simulink model "TV_2018_HIL"  (R2016a)
settings: Solver=FixedStepAuto  StartTime=0.0  StopTime=inf  FixedStep=0.001  RelTol=1e-3
PreLoadFcn:
  | TV_2017_parameters
values from neighbouring files (symbols this model uses):
  battery_voltage = single(530)    [HIL_parameters.m]    (also in HIL_parameters_2018.m; TV_2017_parameters.m; TV_2017_parameters_VD.m)
  car_params = Simulink_Car_params    [HIL_parameters.m]    (also in HIL_parameters_2018.m; TV_2017_parameters.m; TV_2017_parameters_VD.m)
  i_Diff = 16    [HIL_parameters.m]    (also in HIL_parameters_2018.m; TV_2017_parameters.m)
  Kp = 1    [HIL_parameters.m]    (also in HIL_parameters_2018.m; TV_2017_parameters.m; TV_2017_parameters_VD.m)
  motor_data = struct    [HIL_parameters.m]    (also in HIL_parameters_2018.m; TV_2017_parameters.m)
  powerLimitControl = Simulink_el    [HIL_parameters.m]    (also in HIL_parameters_2018.m; TV_2017_parameters.m; TV_2017_parameters_VD.m)
  settings = Simulink_Settings    [HIL_parameters.m]    (also in HIL_parameters_2018.m; TV_2017_parameters.m; TV_2017_parameters_VD.m)
  SpdC_BCC = 0    [HIL_parameters.m]    (also in HIL_parameters_2018.m; TV_2017_parameters.m; TV_2017_parameters_VD.m)
  Speed_Neg_sat = -21    [HIL_parameters.m]    (also in HIL_parameters_2018.m; TV_2017_parameters.m; TV_2017_parameters_VD.m)
  Speed_Pos_sat = 21    [HIL_parameters.m]    (also in HIL_parameters_2018.m; TV_2017_parameters.m; TV_2017_parameters_VD.m)
  SteeringAngleFL = [-23.80 -22.65 -21.50 -20.34 -19.18 -18.03 -16.86 -15.70 -14.53 -13.35 -12.18 -10.99 -9.80 -8.61 -7.40 -6.19 -4.97 -3.75 -2.51 -1.26 0 1.27 2.56 3.85 5.17 6.50 7.84 9.21 10.59 12.00 13.42 14.88 16.36 17.87 19.41 20.99 22.61 24.26 25.97 27.73 29.54]    [CarSetupAnalysis2018.m]    (also in HIL_parameters_2018.m; TV_2017_parameters.m; TV_2017_parameters_VD.m = [-24.129 -22.950 -21.772 -20.593 -19.413 -18.232 -17.050 -15)
  SteeringAngleFR = [-29.54 -27.73 -25.97 -24.26 -22.61 -20.99 -19.41 -17.87 -16.36 -14.88 -13.42 -12.00 -10.59 -9.21 -7.84 -6.50 -5.17 -3.85 -2.56 -1.27 0 1.26 2.51 3.75 4.97 6.19 7.40 8.61 9.80 10.99 12.18 13.35 14.53 15.70 16.86 18.03 19.18 20.34 21.50 22.65 23.80]    [CarSetupAnalysis2018.m]    (also in HIL_parameters_2018.m; TV_2017_parameters.m; TV_2017_parameters_VD.m = [-29.3050 -27.5340 -25.8140 -24.1410 -22.5110 -20.9180 -19.3)
  SteeringWhAngle = [-105 -99.75 -94.5 -89.25 -84 -78.75 -73.5 -68.25 -63 -57.75 -52.5 -47.25 -42 -36.75 -31.5 -26.25 -21.0 -15.75 -10.5 -5.25 0.0 5.25 10.50 15.75 21.00 26.25 31.50 36.75 42.00 47.25 52.50 57.75  63.00 68.25 73.50 78.75 84.00 89.25 94.50 99.75 105.00]    [TV_2017_parameters_VD.m]
  Tn_n = 0    [HIL_parameters.m]    (also in HIL_parameters_2018.m; TV_2017_parameters.m; TV_2017_parameters_VD.m)
  tractionControl = Simulink_tc    [HIL_parameters.m]    (also in HIL_parameters_2018.m; IterativeTractionControlTuning.m; TV_2017_parameters.m; TV_2017_parameters_VD.m)
  yawMomentGenerator = struct    [HIL_parameters.m]    (also in HIL_parameters_2018.m = Simulink_yawRate2; TV_2017_parameters.m = Simulink_yawRate2)
  yawRateControl = Simulink_yawRate    [HIL_parameters.m]    (also in HIL_parameters_2018.m; TV_2017_parameters.m; TV_2017_parameters_VD.m)
undefined symbols (not defined in the file or in its folder): canChannel, DiscIntNeverNeededParam, magnitude, speedEstimation, TC_Decr_Gas, TC_Derivative, TC_Incr_Gas, TC_On, TC_Relay_Off, TC_Relay_On
libraries: CarMaker4SL x366, simulink_extras x63, canmsglib x55, canlib x41, simulink x37, dspfdesign x2, sldrtlib x1
(part 1 of 15)
settings Model: Creator=fh  LastModifiedBy=95fre
settings DataIOCC: LimitDataPoints=on  SaveFormat=Array  SignalLoggingSaveFormat=ModelDataLogs  SignalLoggingName=sigsOut
settings OptimizationCC: DefaultUnderspecifiedDataType=single  OptimizeBlockIOStorage=off  BufferReuse=off  GlobalBufferReuse=off  ExpressionFolding=off  ExpressionDepthLimit=2147483647  LocalBlockOutputs=off  OptimizeModelRefInitCode=on  LifeSpan=Inf  MaxStackSize=64
settings DebuggingCC: SaveWithParameterizedLinksMsg=none  UnderspecifiedInitializationDetection=Classic  SignalResolutionControl=TryResolveAllWithWarning  MultiTaskDSMMsg=warning  MultiTaskCondExecSysMsg=none  BusObjectLabelMismatch=error  ModelReferenceVersionMismatchMessage=warning  StateNameClashWarn=warning
settings HardwareCC: ProdBitPerPointer=32  ProdLargestAtomicInteger=Long  ProdLargestAtomicFloat=Double  ProdWordSize=32  ProdHWDeviceType=ARM Compatible->ARM Cortex  TargetLargestAtomicInteger=Long  TargetLargestAtomicFloat=Double  TargetEndianess=LittleEndian  TargetHWDeviceType=ARM Compatible->ARM Cortex
settings ModelReferenceCC: PropagateSignalLabelsOutOfModel=off
settings RTWCC: SystemTargetFile=ert.tlc  GenCodeOnly=on  TemplateMakefile=ert_default_tmf  GenerateReport=on  Toolchain=GNU Tools for ARM Embedded Processors  BuildConfiguration=Debug  IncludeHyperlinkInReport=on  LaunchReport=on
settings CodeAppCC: ForceParamTrailComments=on  IgnoreCustomStorageClasses=off  SimulinkDataObjDesc=on  SFDataObjDesc=on  MATLABFcnDesc=on  InsertBlockDesc=on  MATLABSourceComments=on  EnableCustomComments=on  ReqsInCode=on
settings ERTTargetCC: GenerateSampleERTMain=on  IncludeMdlTerminateFcn=off  MatFileLogging=on  SupportNonFinite=off  SupportComplex=off  SupportVariableSizeSignals=on  ERTCustomFileTemplate=example_file_process.tlc  SuppressUnreachableDefaultCases=off
settings ConfigComp: CovHTMLOptions=-sRT=1 -sVT=0 -aTS=1 -bRG=1 -bTC=1 -hTR=0 -nFC=0 -nFD=1 -scm=1 -bcm=1 -xEv=0 -xEM=0  CovModelRefEnable=Off  PSAutoStubLUT=off

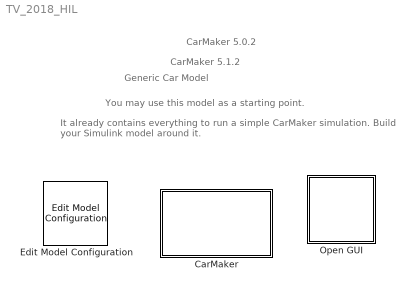
== system TV_2018_HIL ==
  note: Generic Car Model
  note: You may use this model as a starting point.
  note: It already contains everything to run a simple CarMaker simulation.
      | Build your Simulink model around it.
  note: CarMaker 5.0.2
  note: CarMaker 5.1.2
  CarMaker : Subsystem  TreatAsAtomicUnit=on
      mask Display: image(imread('CarMakerSys.png'));
  Edit Model Configuration : CarMaker4SL/Edit Model Configuration
  Open GUI : Subsystem  LoadFcn=if ~length(which('cmcmd')), cmenv; end
      settings: OpenFcn=cmblockmagic('gui_fix_display'); CM_Simulink
      mask Display: image('CarMakerGUI.png');

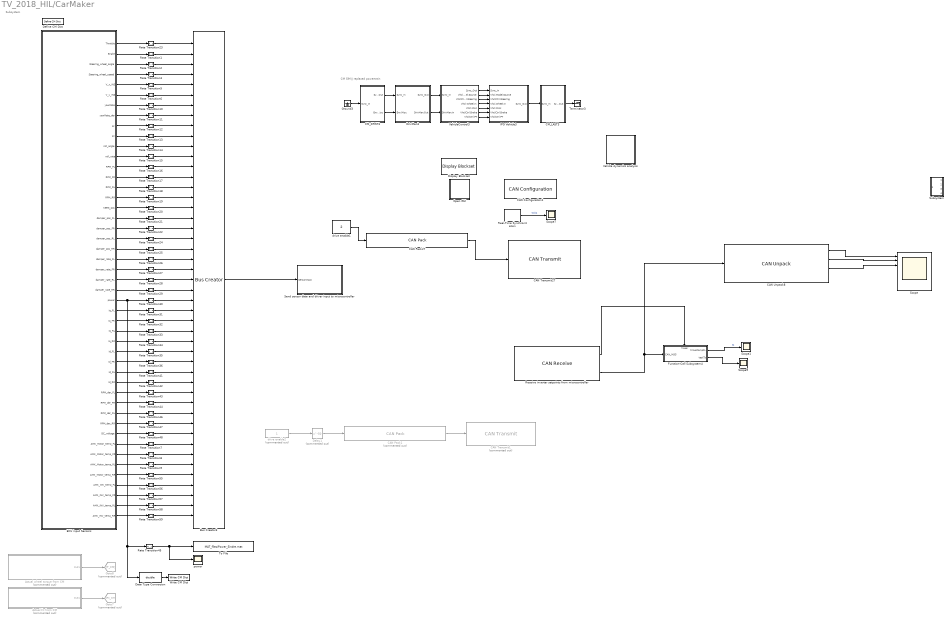
== system TV_2018_HIL/CarMaker ==
  note: Subsystem
  note: CM SIM|| replaced powertrain
  Actual Fz from CM : Subsystem  Commented=on
  Actual wheel torque from CM : Subsystem  Commented=on
  Bus Creator3 : BusCreator  Inputs=47  OutDataTypeStr=Bus: SensorInputs  NonVirtualBus=on
      settings: InheritFromInputs=off
  CAN Configuration1 : canlib/CAN Configuration  BlockHandle=108.0002  DeviceMenu=Kvaser Virtual 1 (Channel 1)  Device=PEAK-System PCAN-USB (PCAN_USBBUS1)  ObjConstructor=canChannel('PEAK-System', 'PCAN_PCIBUS1')  BusSpeed=1000000  EnableBitParameters=off  SJW=NaN  TSEG1=NaN  TSEG2=NaN  NSamples=NaN  AckMode=Normal
  CAN Pack1 : canmsglib/CAN Pack  Commented=on  MsgList=(none)  MsgName=CAN Msg  MsgIDType=Standard (11-bit identifier)  MsgIdentifier=DRIVE_ENABLE  MsgLength=0  NSignals=0  StartBits=0  SignalSizes=0  ByteOrders=0  DataTypes=0  MultiplexTypes=0  MultiplexValues=0  Factors=0  Offsets=0  Minimums=0  Maximums=0  Remote=off
      settings: DataFormat=manually specified signals
  CAN Pack27 : canmsglib/CAN Pack  MsgList=(none)  MsgName=CAN Msg  MsgIDType=Standard (11-bit identifier)  MsgIdentifier=BMS_STATE  MsgLength=4  NSignals=0  StartBits=0  SignalSizes=0  ByteOrders=0  DataTypes=0  MultiplexTypes=0  MultiplexValues=0  Factors=0  Offsets=0  Minimums=0  Maximums=0  Remote=off
      settings: DataFormat=raw data
  CAN Transmit1 : canlib/CAN Transmit  Commented=on  BlockHandle=111.0002  DeviceMenu=Kvaser Virtual 1 (Channel 1)  Device=PEAK-System PCAN-USB (PCAN_USBBUS1)  ObjConstructor=canChannel('PEAK-System', 'PCAN_PCIBUS1')  EnablePeriodicTransmit=off  MessagePeriod=1.000
  CAN Transmit27 : canlib/CAN Transmit  BlockHandle=112.0002  DeviceMenu=Kvaser Virtual 1 (Channel 1)  Device=PEAK-System PCAN-USB (PCAN_USBBUS1)  ObjConstructor=canChannel('PEAK-System', 'PCAN_PCIBUS1')  EnablePeriodicTransmit=off  MessagePeriod=1.000
  CAN Unpack8 : canmsglib/CAN Unpack  MsgList=(none)  MsgName=TestTimestamp  MsgIDType=Standard (11-bit identifier)  MsgIdentifier=ECU_STATE  MsgLength=4  SignalInfo=sys_state$0$16$1$2$1$0$1$0$-Inf$Inf$#Torque_Alloc$16$8$1$2$1$0$1$0$-Inf$Inf$#Vehicle_state$24$8$1$2$1$0$1$0$-Inf$Inf$#  NSignals=3  IDPort=off  TimestampPort=on  ErrorPort=off  RemotePort=off  LengthPort=off  StatusPort=off  StartBits=str2num('[int32(0);int32(16);int32(24)]')  SignalSizes=str2num('[int32(16);int32(8);int32(8)]')  ByteOrders=str2num('[int32(1);int32(1);int32(1)]')  DataTypes=str2num('[int32(2);int32(2);int32(2)]')  MultiplexTypes=str2num('[int32(1);int32(1);int32(1)]')  MultiplexValues=str2num('[double(0);double(0);double(0)]')  Factors=str2num('[double(1);double(1);double(1)]')  Offsets=str2num('[double(0);double(0);double(0)]')  Minimums=str2num('[double(-Inf);double(-Inf);double(-Inf)]')  Maximums=str2num('[double(Inf);double(Inf);double(Inf)]')
  CM_FIRST3 : Subsystem
  CM_LAST3 : Subsystem
  Data Type Conversion : DataTypeConversion  OutDataTypeStr=double
  Define CM Dict : CarMaker4SL/Define CM Dict  xname=Power  xmono=off  xtype=Double  xdvaplace=None  xnstates=0  xfirststate=0  xinitial=0
  Delay1 : Delay  Commented=on  DelayLength=50
  Display Blockset : CarMaker4SL/Display Blockset
  DrivMan3 : Subsystem
  "ECU input Sensors " : Subsystem  SystemSampleTime=settings.control_system_sample_time
  Function-Call Subsystem4 : Subsystem  TreatAsAtomicUnit=on
  Goto7 : Goto  Commented=on  GotoTag=Fz_CM
  Goto8 : Goto  Commented=on  GotoTag=T_CM
  Ground3 : Ground
  IPG Vehicle3 : Subsystem  TreatAsAtomicUnit=on
  Open GUI : Subsystem  LoadFcn=if ~length(which('cmcmd')), cmenv; end
      settings: OpenFcn=cmblockmagic('gui_fix_display'); CM_Simulink
      mask Display: image('CarMakerGUI.png');
  Rate Transition{1..3,5..36,41..48,55..59} (48 alike) : RateTransition  OutPortSampleTime=matlab_params.sensor_sampling_time
  Real-Time Synchronization : sldrtlib/Real-Time Synchronization  SampleTime=0.01  MaxMissedTicks=100000  ShowMissedTicks=on  YieldWhenWaiting=on
  Receive inverter setpoints from microcontroller : canlib/CAN Receive  BlockHandle=19018.001  DeviceMenu=Kvaser Virtual 1 (Channel 1)  Device=PEAK-System PCAN-USB (PCAN_USBBUS1)  ObjConstructor=canChannel('PEAK-System', 'PCAN_PCIBUS1')  EnableStandardIDsFilter=off  StandardIDs=listen_ID  EnableExtendedIDsFilter=off  ExtendedIDs=0  SampleTime=0.001  MsgsPerTimestep=all  StdIDsCombo=Allow all  ExtIDsCombo=Allow all  InternalFilterUpdateStatus=on
  Scope : Scope  NumInputPorts=8
  Scope1 : Scope
  Scope7 : Scope
  Scope9 : Scope
  "Send sensor data and driver input to microcontroller " : Subsystem
  Subsystem : Subsystem
  Terminator3 : Terminator
  To File : ToFile  Filename=MAT_files\Power_Sindre.mat  MatrixName=Power  SaveFormat=Timeseries
  Vehicle dynamics analysis : Subsystem
  VehicleControl3 : Subsystem
  Write CM Dict : CarMaker4SL/Write CM Dict  xname=Power  xsync=off
  drive enable1 : Constant  Value=2  OutDataTypeStr=uint8
  drive enable2 : Constant  Commented=on
  power : Scope
  wires:
  VehicleControl3/7(VhclCtrl.PT) -> IPG Vehicle3/7(VhclCtrl.PT)
  VehicleControl3/6(VhclCtrl.Brake) -> IPG Vehicle3/6(VhclCtrl.Brake)
  CM_FIRST3/1(Sync_Out) -> DrivMan3/1(Sync_In)
  CM_FIRST3/2(Env.Misc) -> DrivMan3/2(Env.Misc)
  VehicleControl3/3(VhclCtrl.Steering) -> IPG Vehicle3/3(VhclCtrl.Steering)
  DrivMan3/2(DrivMan.Out) -> VehicleControl3/2(DrivMan.In)
  VehicleControl3/2(Vhcl.Model.Source) -> IPG Vehicle3/2(Vhcl.Model.Source)
  VehicleControl3/5(Vhcl.Misc) -> IPG Vehicle3/5(Vhcl.Misc)
  VehicleControl3/1(Sync_Out) -> IPG Vehicle3/1(Sync_In)
  VehicleControl3/4(Vhcl.Wheel.In) -> IPG Vehicle3/4(Vhcl.Wheel.In)
  DrivMan3/1(Sync_Out) -> VehicleControl3/1(Sync_In)
  Ground3/1 -> CM_FIRST3/1(Sync_In)
  IPG Vehicle3/1(Sync_Out) -> CM_LAST3/1(Sync_In)
  CM_LAST3/1(Sync_Out) -> Terminator3/1
  Receive inverter setpoints from microcontroller/1 -> Function-Call Subsystem4/Trigger
  Function-Call Subsystem4/1(timestampFL) -> Scope1/1  "ts"
  Function-Call Subsystem4/2(testTs) -> Scope9/1
  Real-Time Synchronization/1 -> Scope7/1  "ticks"
  Rate Transition9/1 -> Bus Creator3/42
  Rate Transition7/1 -> Bus Creator3/40
  Rate Transition27/1 -> Bus Creator3/23
  "ECU input Sensors "/40(AMK_Motor_temp_FL) -> Rate Transition7/1
  "ECU input Sensors "/46(AMK_INV_temp_RL) -> Rate Transition58/1
  "ECU input Sensors "/41(AMK_Motor_temp_FR) -> Rate Transition8/1
  Rate Transition10/1 -> Bus Creator3/7
  Rate Transition46/1 -> Bus Creator3/37
  "ECU input Sensors "/44(AMK_INV_temp_FL) -> Rate Transition56/1
  Rate Transition5/1 -> Bus Creator3/5
  Actual Fz from CM/1(Out1) -> Goto7/1
  "ECU input Sensors "/42(AMK_Motor_temp_RL) -> Rate Transition9/1
  "ECU input Sensors "/26(power) -> Data Type Conversion/1, Rate Transition45/1, Rate Transition30/1
  Rate Transition58/1 -> Bus Creator3/46
  Rate Transition32/1 -> Bus Creator3/28
  Rate Transition57/1 -> Bus Creator3/45
  Rate Transition47/1 -> Bus Creator3/38
  "ECU input Sensors "/43(AMK_Motor_temp_RR) -> Rate Transition55/1
  Rate Transition48/1 -> Bus Creator3/39
  Rate Transition19/1 -> Bus Creator3/16
  Actual wheel torque from CM/1(Out1) -> Goto8/1
  Rate Transition13/1 -> Bus Creator3/10
  Rate Transition59/1 -> Bus Creator3/47
  Rate Transition56/1 -> Bus Creator3/44
  "ECU input Sensors "/47(AMK_INV_temp_RR) -> Rate Transition59/1
  Rate Transition55/1 -> Bus Creator3/43
  Rate Transition33/1 -> Bus Creator3/29
  "ECU input Sensors "/45(AMK_INV_temp_FR) -> Rate Transition57/1
  Data Type Conversion/1 -> Write CM Dict/1
  Rate Transition41/1 -> Bus Creator3/33
  Rate Transition34/1 -> Bus Creator3/30
  Rate Transition43/1 -> Bus Creator3/35
  Rate Transition42/1 -> Bus Creator3/34
  Rate Transition44/1 -> Bus Creator3/36
  Rate Transition8/1 -> Bus Creator3/41
  Rate Transition36/1 -> Bus Creator3/32
  Rate Transition35/1 -> Bus Creator3/31
  Rate Transition6/1 -> Bus Creator3/6
  Rate Transition28/1 -> Bus Creator3/24
  Rate Transition21/1 -> Bus Creator3/18
  "ECU input Sensors "/32(Id_FR) -> Rate Transition36/1
  "ECU input Sensors "/3("Steering_wheel_angle ") -> Rate Transition2/1
  "ECU input Sensors "/34(Id_RR) -> Rate Transition42/1
  "ECU input Sensors "/7(yawRate) -> Rate Transition10/1
  "ECU input Sensors "/31(Id_FL) -> Rate Transition35/1
  "ECU input Sensors "/1("Throttle ") -> Rate Transition23/1
  Rate Transition26/1 -> Bus Creator3/22
  Rate Transition31/1 -> Bus Creator3/27
  "ECU input Sensors "/13(RPM_FL) -> Rate Transition16/1
  Rate Transition18/1 -> Bus Creator3/15
  Rate Transition11/1 -> Bus Creator3/8
  Rate Transition14/1 -> Bus Creator3/11
  Rate Transition30/1 -> Bus Creator3/26
  "ECU input Sensors "/16(RPM_RR) -> Rate Transition19/1
  Rate Transition23/1 -> Bus Creator3/1
  "ECU input Sensors "/6(V_y_INS) -> Rate Transition6/1
  "ECU input Sensors "/24(damper_rate_RL) -> Rate Transition28/1
  "ECU input Sensors "/19(damper_pos_FR) -> Rate Transition22/1
  "ECU input Sensors "/29(Iq_RL) -> Rate Transition33/1
  "ECU input Sensors "/25(damper_rate_RR) -> Rate Transition29/1
  "ECU input Sensors "/5(V_x_INS) -> Rate Transition5/1
  Rate Transition2/1 -> Bus Creator3/3
  Rate Transition17/1 -> Bus Creator3/14
  "ECU input Sensors "/30(Iq_RR) -> Rate Transition34/1
  "ECU input Sensors "/12(roll_rate) -> Rate Transition15/1
  "ECU input Sensors "/22(damper_rate_FL) -> Rate Transition26/1
  "ECU input Sensors "/28(Iq_FR) -> Rate Transition32/1
  "ECU input Sensors "/11(roll_angle) -> Rate Transition14/1
  "ECU input Sensors "/2("Brake ") -> Rate Transition1/1
  "ECU input Sensors "/17(KERS_pos) -> Rate Transition20/1
  Rate Transition15/1 -> Bus Creator3/12
  Rate Transition29/1 -> Bus Creator3/25
  Rate Transition24/1 -> Bus Creator3/20
  Rate Transition1/1 -> Bus Creator3/2
  Rate Transition20/1 -> Bus Creator3/17
  Rate Transition12/1 -> Bus Creator3/9
  "ECU input Sensors "/20(damper_pos_RL) -> Rate Transition24/1
  "ECU input Sensors "/15(RPM_RL) -> Rate Transition18/1
  Rate Transition22/1 -> Bus Creator3/19
  Rate Transition3/1 -> Bus Creator3/4
  Rate Transition25/1 -> Bus Creator3/21
  "ECU input Sensors "/10("ax ") -> Rate Transition13/1
  Rate Transition16/1 -> Bus Creator3/13
  "ECU input Sensors "/39(DC_voltage) -> Rate Transition48/1
  "ECU input Sensors "/18(damper_pos_FL) -> Rate Transition21/1
  "ECU input Sensors "/8(yawRate_der) -> Rate Transition11/1
  "ECU input Sensors "/4(Steering_wheel_speed) -> Rate Transition3/1
  "ECU input Sensors "/27(Iq_FL) -> Rate Transition31/1
  "ECU input Sensors "/14(RPM_FR) -> Rate Transition17/1
  "ECU input Sensors "/21(damper_pos_RR) -> Rate Transition25/1
  "ECU input Sensors "/9(ay) -> Rate Transition12/1
  "ECU input Sensors "/33(Id_RL) -> Rate Transition41/1
  "ECU input Sensors "/23(damper_rate_FR) -> Rate Transition27/1
  Rate Transition45/1 -> power/1, To File/1
  "ECU input Sensors "/35(RPM_der_FL) -> Rate Transition43/1
  "ECU input Sensors "/36(RPM_der_FR) -> Rate Transition44/1
  "ECU input Sensors "/38(RPM_der_RR) -> Rate Transition47/1
  "ECU input Sensors "/37(RPM_der_RL) -> Rate Transition46/1
  CAN Pack27/1 -> CAN Transmit27/1
  Receive inverter setpoints from microcontroller/2 -> CAN Unpack8/1, Function-Call Subsystem4/1(CAN_MSG)
  CAN Unpack8/1 -> Scope/1
  CAN Unpack8/2 -> Scope/2
  CAN Unpack8/3 -> Scope/3
  drive enable1/1 -> CAN Pack27/1
  CAN Pack1/1 -> CAN Transmit1/1
  drive enable2/1 -> Delay1/1
  Delay1/1 -> CAN Pack1/1
  Bus Creator3/1 -> "Send sensor data and driver input to microcontroller "/1(SensorInput)

== system TV_2018_HIL/Open GUI ==
  S-Function : S-Function  FunctionName=cm_gui  SFunctionDeploymentMode=off  EnableBusSupport=off

== system TV_2018_HIL/CarMaker/Actual Fz from CM ==
  Bus Creator1 : BusCreator  Inputs=4
  Bus Creator4 : BusCreator  Inputs=4  OutDataTypeStr=Bus: normalForces  NonVirtualBus=on
      settings: InheritFromInputs=off
  Data Type Conversion{4..11} (8 alike) : DataTypeConversion  OutDataTypeStr=single
  Divide{,1..3} (4 alike) : Product  Inputs=*/
  Friction : Scope
  Rate Transition4 : RateTransition  OutPortSampleTime=matlab_params.sensor_sampling_time
  Read CM Dict10 : CarMaker4SL/Read CM Dict  xname=Vhcl.RL.Fx  xsync=off
  Read CM Dict11 : CarMaker4SL/Read CM Dict  xname=Vhcl.RR.Fx  xsync=off
  Read CM Dict3 : CarMaker4SL/Read CM Dict  xname=Vhcl.FR.Fz  xsync=off
  Read CM Dict4 : CarMaker4SL/Read CM Dict  xname=Vhcl.FL.Fz  xsync=off
  Read CM Dict5 : CarMaker4SL/Read CM Dict  xname=Vhcl.RR.Fz  xsync=off
  Read CM Dict6 : CarMaker4SL/Read CM Dict  xname=Vhcl.RL.Fz  xsync=off
  Read CM Dict8 : CarMaker4SL/Read CM Dict  xname=Vhcl.FL.Fx  xsync=off
  Read CM Dict9 : CarMaker4SL/Read CM Dict  xname=Vhcl.FR.Fx  xsync=off
  Out1 : Outport
  wires:
  Rate Transition4/1 -> Out1/1
  Read CM Dict4/1 -> Data Type Conversion4/1
  Read CM Dict5/1 -> Data Type Conversion7/1
  Read CM Dict3/1 -> Data Type Conversion5/1
  Read CM Dict6/1 -> Data Type Conversion6/1
  Data Type Conversion7/1 -> Bus Creator4/4, Divide3/2
  Data Type Conversion5/1 -> Bus Creator4/2, Divide1/2
  Data Type Conversion6/1 -> Bus Creator4/3, Divide2/2
  Divide/1 -> Bus Creator1/1  "FL"
  Read CM Dict10/1 -> Data Type Conversion10/1
  Data Type Conversion11/1 -> Divide3/1
  Data Type Conversion9/1 -> Divide1/1
  Data Type Conversion8/1 -> Divide/1
  Read CM Dict9/1 -> Data Type Conversion9/1
  Read CM Dict11/1 -> Data Type Conversion11/1
  Divide3/1 -> Bus Creator1/4  "RR"
  Bus Creator1/1 -> Friction/1
  Data Type Conversion4/1 -> Bus Creator4/1, Divide/2
  Read CM Dict8/1 -> Data Type Conversion8/1
  Divide2/1 -> Bus Creator1/3  "RL"
  Bus Creator4/1 -> Rate Transition4/1
  Data Type Conversion10/1 -> Divide2/1
  Divide1/1 -> Bus Creator1/2  "FR"

== system TV_2018_HIL/CarMaker/Actual wheel torque from CM ==
  Bus Creator2 : BusCreator  Inputs=4  OutDataTypeStr=Bus: T_meas
      settings: InheritFromInputs=off
  Data Type Conversion{1..3,12..15} (7 alike) : DataTypeConversion  OutDataTypeStr=single
  Rate Transition{37..40} (4 alike) : RateTransition  OutPortSampleTime=matlab_params.sensor_sampling_time
  Read CM Dict1 : CarMaker4SL/Read CM Dict  xname=Car.DampFL.Frc_tot  xsync=off
  Read CM Dict12 : CarMaker4SL/Read CM Dict  xname=PT.WFL.Trq_Drive  xsync=off
  Read CM Dict2 : CarMaker4SL/Read CM Dict  xname=Car.SpringFL.Frc_tot  xsync=off
  Read CM Dict45 : CarMaker4SL/Read CM Dict  xname=PT.WFR.Trq_Drive  xsync=off
  Read CM Dict46 : CarMaker4SL/Read CM Dict  xname=PT.WRL.Trq_Drive  xsync=off
  Read CM Dict47 : CarMaker4SL/Read CM Dict  xname=PT.WRR.Trq_Drive  xsync=off
  Read CM Dict7 : CarMaker4SL/Read CM Dict  xname=Car.StabiFL.Frc_tot  xsync=off
  "damp force fl " : Scope
  spring force fl : Scope
  spring force fl1 : Scope
  Out1 : Outport
  wires:
  Bus Creator2/1 -> Out1/1
  Rate Transition38/1 -> Bus Creator2/2
  Data Type Conversion1/1 -> "damp force fl "/1
  Data Type Conversion2/1 -> spring force fl/1
  Data Type Conversion3/1 -> spring force fl1/1
  Read CM Dict2/1 -> Data Type Conversion2/1
  Read CM Dict7/1 -> Data Type Conversion3/1
  Read CM Dict1/1 -> Data Type Conversion1/1
  Data Type Conversion12/1 -> Rate Transition37/1  "FL"
  Data Type Conversion14/1 -> Rate Transition39/1  "RL"
  Read CM Dict46/1 -> Data Type Conversion14/1
  Rate Transition39/1 -> Bus Creator2/3
  Data Type Conversion15/1 -> Rate Transition40/1  "RR"
  Read CM Dict12/1 -> Data Type Conversion12/1
  Read CM Dict47/1 -> Data Type Conversion15/1
  Rate Transition37/1 -> Bus Creator2/1
  Rate Transition40/1 -> Bus Creator2/4
  Read CM Dict45/1 -> Data Type Conversion13/1
  Data Type Conversion13/1 -> Rate Transition38/1  "FR"

== system TV_2018_HIL/CarMaker/CM_FIRST3 ==
  Sync_In : Inport
  BusCreator1 : BusCreator  Inputs=8
  BusCreator2 : BusCreator  Inputs=6
  Demux1 : Demux  Outputs=14
  Environment : S-Function  FunctionName=CM_Sfun  Parameters='Environment'  SFunctionDeploymentMode=off  EnableBusSupport=off
  IoIn : S-Function  FunctionName=CM_Sfun  Parameters='IoIn'  SFunctionDeploymentMode=off  EnableBusSupport=off
  Terminator : Terminator
  Sync_Out : Outport
  Env.Misc : Outport  Port=2
  wires:
  BusCreator2/1 -> Terminator/1  "IF Environment (in)"
  BusCreator1/1 -> Env.Misc/1
  Demux1/14 -> BusCreator2/6  "Env sRoad"
  Demux1/13 -> BusCreator2/5  "Env PoI_GCS Elev"
  Demux1/12 -> BusCreator2/4  "Env PoI_GCS Lat"
  Demux1/11 -> BusCreator2/3  "Env PoI_GCS Long"
  Demux1/10 -> BusCreator2/2  "Env Time"
  Demux1/9 -> BusCreator2/1  "Env yDay"
  Demux1/8 -> BusCreator1/8  "Env WindVel_tot z"
  Demux1/7 -> BusCreator1/7  "Env WindVel_tot y"
  Demux1/6 -> BusCreator1/6  "Env WindVel_tot x"
  Demux1/5 -> BusCreator1/5  "Env SolarRadiation"
  Demux1/4 -> BusCreator1/4  "Env AirHumidity"
  Demux1/3 -> BusCreator1/3  "Env AirPressure"
  Demux1/2 -> BusCreator1/2  "Env AirDensity"
  Demux1/1 -> BusCreator1/1  "Env Temperature"
  Environment/2 -> Demux1/1
  Environment/1 -> Sync_Out/1
  IoIn/1 -> Environment/1
  Sync_In/1 -> IoIn/1

== system TV_2018_HIL/CarMaker/CM_LAST3 ==
  Sync_In : Inport
  CM_User : S-Function  FunctionName=CM_Sfun  Parameters='CM_User'  SFunctionDeploymentMode=off  EnableBusSupport=off
  IoOut : S-Function  FunctionName=CM_Sfun  Parameters='IoOut'  SFunctionDeploymentMode=off  EnableBusSupport=off
  Sync_Out : Outport
  wires:
  IoOut/1 -> Sync_Out/1
  CM_User/1 -> IoOut/1
  Sync_In/1 -> CM_User/1

== system TV_2018_HIL/CarMaker/DrivMan3 ==
  note: There's rarely a reason to override DrivMan signals.
      | Use the VehicleControl interface for this purpose.
  Sync_In : Inport
  Env.Misc : Inport  Port=2
  BusCreator : BusCreator  Inputs=17
  Demux : Demux  Outputs=17
  DrivMan : S-Function  FunctionName=CM_Sfun  Parameters='DrivMan'  SFunctionDeploymentMode=off  EnableBusSupport=off
  Sync_Out : Outport
  DrivMan.Out : Outport  Port=2
  wires:
  Demux/17 -> BusCreator/17  "DrivMan Steering Trq"
  Demux/16 -> BusCreator/16  "DrivMan Steering AngAcc"
  Demux/15 -> BusCreator/15  "DrivMan Steering AngVel"
  Demux/14 -> BusCreator/14  "DrivMan Steering Ang"
  Demux/13 -> BusCreator/13  "DrivMan Gas"
  Demux/12 -> BusCreator/12  "DrivMan Clutch"
  Demux/11 -> BusCreator/11  "DrivMan BrakePark"
  Demux/10 -> BusCreator/10  "DrivMan Brake"
  Demux/9 -> BusCreator/9  "DrivMan GearNo"
  Demux/8 -> BusCreator/8  "DrivMan SelectorCtrl"
  Demux/7 -> BusCreator/7  "DrivMan UserSignal4"
  Demux/6 -> BusCreator/6  "DrivMan UserSignal3"
  Demux/5 -> BusCreator/5  "DrivMan UserSignal2"
  Demux/4 -> BusCreator/4  "DrivMan UserSignal1"
  Demux/3 -> BusCreator/3  "DrivMan UserSignal0"
  Demux/2 -> BusCreator/2  "DrivMan Key"
  Demux/1 -> BusCreator/1  "DrivMan SST"
  Env.Misc/1 -> DrivMan/2
  Sync_In/1 -> DrivMan/1
  DrivMan/1 -> Sync_Out/1
  BusCreator/1 -> DrivMan.Out/1
  DrivMan/2 -> Demux/1

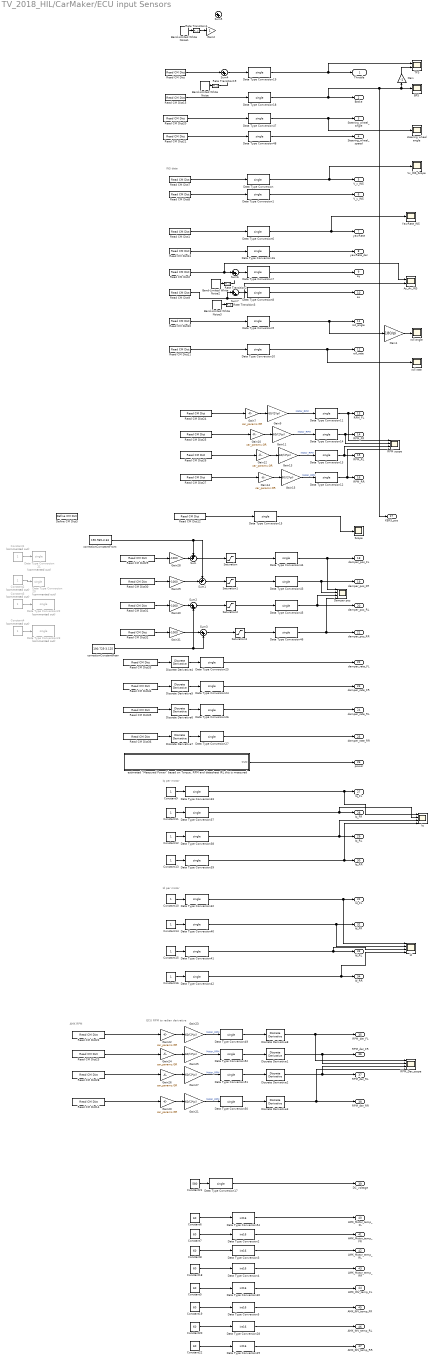
== system TV_2018_HIL/CarMaker/ECU input Sensors  ==
  note: INS data
  note: ECU RPM to radian derivative
  note: AMK RPM
  note: Id per motor
  note: Iq per motor
  Ay_Ax_INS : Scope  NumInputPorts=2
  BPS : Scope
  Band-Limited White Noise : simulink/Sources/Band-Limited White Noise  Cov=[0.00002]  Ts=0.1  seed=[23341]
  Band-Limited White Noise1 : simulink/Sources/Band-Limited White Noise  Cov=[0.00002]  Ts=0.1  seed=[23341]
  Band-Limited White Noise2 : simulink/Sources/Band-Limited White Noise  Cov=[0.01]  Ts=0.1  seed=[23341]
  Band-Limited White Noise3 : simulink/Sources/Band-Limited White Noise  Cov=[0.01]  Ts=0.1  seed=[23341]
  Constant{1..4} (4 alike) : Constant  Commented=on
  Constant{9..16} (8 alike) : Constant
  Constant{5..8,18..20,22} (8 alike) : Constant  Value=60
  Constant21 : Constant  Value=580
  Damper pos : Scope  NumInputPorts=4
  Data Type Conversion{,1,6..19,24..27,32..33,37..52} (38 alike) : DataTypeConversion  OutDataTypeStr=single
  Data Type Conversion{2..5,28..30,54} (8 alike) : DataTypeConversion  OutDataTypeStr=int16
  Data Type Conversion{20..23} (4 alike) : DataTypeConversion  Commented=on  OutDataTypeStr=single
  Define CM Dict3 : CarMaker4SL/Define CM Dict  xname=KERS_pos  xmono=off  xtype=Double  xdvaplace=None  xnstates=0  xfirststate=0  xinitial=0
  Discrete Derivative{1..3,8} (4 alike) : simulink/Discrete/Discrete Derivative  gainval=1.0  ICPrevScaledInput=0.0  InputProcessing=Inherited  OutMin=[]  OutMax=[]  OutDataType=fixdt(1, 16)  OutScaling=2^-10  DoSatur=off
  Discrete Derivative{4..7} (4 alike) : simulink/Discrete/Discrete Derivative  gainval=1.0  ICPrevScaledInput=0.0  OutMin=[]  OutMax=[]  OutDataType=fixdt(1, 16)  OutScaling=2^-10  DoSatur=off
  Gain : Gain  Gain=-1
  Gain1 : Gain  Gain=180/pi
  Gain{7,10,12,14,20,22,24,26} (8 alike) : Gain  Gain=car_params.GR
  Gain{9,11,13,15,21,23,25,27} (8 alike) : Gain  Gain=60/(2*pi)
  Gain2 : Gain
  Gain{28..31} (4 alike) : Gain  Gain=-1000
  Id : Scope  NumInputPorts=4
  Iq : Scope  NumInputPorts=4
  RPM scope : Scope  NumInputPorts=4
  "RPM_Der_scope " : Scope  NumInputPorts=4
  Rate Transition{1..3,19} (4 alike) : RateTransition  OutPortSampleTimeOpt=Inherit  OutPortSampleTime=matlab_params.sensor_sampling_time
  Read CM Dict : CarMaker4SL/Read CM Dict  xname=VC.Gas  xsync=off
  Read CM Dict1 : CarMaker4SL/Read CM Dict  xname=Vhcl.YawRate  xsync=off
  Read CM Dict10 : CarMaker4SL/Read CM Dict  xname=Vhcl.Roll  xsync=off
  Read CM Dict11 : CarMaker4SL/Read CM Dict  xname=Vhcl.RollVel  xsync=off
  Read CM Dict12 : CarMaker4SL/Read CM Dict  xname=KERS_pos  xsync=off
  Read CM Dict13 : CarMaker4SL/Read CM Dict  xname=Vhcl.YawAcc  xsync=off
  Read CM Dict14 : CarMaker4SL/Read CM Dict  xname=Car.WheelSpd_RR  xsync=off
  Read CM Dict15 : CarMaker4SL/Read CM Dict  xname=VC.Brake  xsync=off
  Read CM Dict2 : CarMaker4SL/Read CM Dict  xname=Car.ay  xsync=off
  Read CM Dict20 : CarMaker4SL/Read CM Dict  xname=Vhcl.Steer.Ang  xsync=off
  Read CM Dict21 : CarMaker4SL/Read CM Dict  xname=Vhcl.Steer.Vel  xsync=off
  Read CM Dict22 : CarMaker4SL/Read CM Dict  xname=Car.WheelSpd_FL  xsync=off
  Read CM Dict23 : CarMaker4SL/Read CM Dict  xname=Car.WheelSpd_FR  xsync=off
  Read CM Dict24 : CarMaker4SL/Read CM Dict  xname=Car.WheelSpd_FL  xsync=off
  Read CM Dict25 : CarMaker4SL/Read CM Dict  xname=Car.WheelSpd_FR  xsync=off
  Read CM Dict26 : CarMaker4SL/Read CM Dict  xname=Car.WheelSpd_RL  xsync=off
  Read CM Dict27 : CarMaker4SL/Read CM Dict  xname=Car.WheelSpd_RR  xsync=off
  Read CM Dict28 : CarMaker4SL/Read CM Dict  xname=Car.WheelSpd_RL  xsync=off
  Read CM Dict29 : CarMaker4SL/Read CM Dict  xname=Car.SpringFL.l  xsync=off
  Read CM Dict30 : CarMaker4SL/Read CM Dict  xname=Car.SpringFR.l  xsync=off
  Read CM Dict31 : CarMaker4SL/Read CM Dict  xname=Car.SpringRL.l  xsync=off
  Read CM Dict32 : CarMaker4SL/Read CM Dict  xname=Car.SpringRR.l  xsync=off
  Read CM Dict33 : CarMaker4SL/Read CM Dict  xname=Car.SpringFL.l  xsync=off
  Read CM Dict34 : CarMaker4SL/Read CM Dict  xname=Car.SpringFR.l  xsync=off
  Read CM Dict35 : CarMaker4SL/Read CM Dict  xname=Car.SpringRL.l  xsync=off
  Read CM Dict36 : CarMaker4SL/Read CM Dict  xname=Car.SpringRR.l  xsync=off
  Read CM Dict7 : CarMaker4SL/Read CM Dict  xname=Car.vx  xsync=off
  Read CM Dict8 : CarMaker4SL/Read CM Dict  xname=Car.vy  xsync=off
  Read CM Dict9 : CarMaker4SL/Read CM Dict  xname=Car.ax  xsync=off
  Saturation{,1..3} (4 alike) : Saturate  UpperLimit=200  LowerLimit=0.001
  Scope : Scope
  Sum : Sum  Inputs=++|
  Sum1 : Sum  Inputs=++|
  Sum{2..7} (6 alike) : Sum  Inputs=|++
  TPS : Scope  NumInputPorts=2
  Vx_INS_Scope : Scope
  YawRate_INS : Scope
  correctionConstantRear : Constant  Value=190.725-3.125
  correctionCornstantFront : Constant  Value=190.965-3.63
  "estimated \"Measured Power\" based on Torque, RPM and datasheet IRL this is measured" : Subsystem
  "roll angle " : Scope
  roll rate : Scope
  steering wheel angle : Scope
  "Throttle " : Outport
  "Brake " : Outport  Port=2
  "Steering_wheel_angle " : Outport  Port=3
  Steering_wheel_speed : Outport  Port=4
  V_x_INS : Outport  Port=5
  V_y_INS : Outport  Port=6
  yawRate : Outport  Port=7
  yawRate_der : Outport  Port=8
  ay : Outport  Port=9
  "ax " : Outport  Port=10
  roll_angle : Outport  Port=11
  roll_rate : Outport  Port=12
  RPM_FL : Outport  Port=13
  RPM_FR : Outport  Port=14
  RPM_RL : Outport  Port=15
  RPM_RR : Outport  Port=16
  KERS_pos : Outport  Port=17
  damper_pos_FL : Outport  Port=18
  damper_pos_FR : Outport  Port=19
  damper_pos_RL : Outport  Port=20
  damper_pos_RR : Outport  Port=21
  damper_rate_FL : Outport  Port=22
  damper_rate_FR : Outport  Port=23
  damper_rate_RL : Outport  Port=24
  damper_rate_RR : Outport  Port=25
  power : Outport  Port=26
  Iq_FL : Outport  Port=27
  Iq_FR : Outport  Port=28
  Iq_RL : Outport  Port=29
  Iq_RR : Outport  Port=30
  Id_FL : Outport  Port=31
  Id_FR : Outport  Port=32
  Id_RL : Outport  Port=33
  Id_RR : Outport  Port=34
  RPM_der_FL : Outport  Port=35
  RPM_der_FR : Outport  Port=36
  RPM_der_RL : Outport  Port=37
  RPM_der_RR : Outport  Port=38
  DC_voltage : Outport  Port=39
  AMK_Motor_temp_FL : Outport  Port=40
  AMK_Motor_temp_FR : Outport  Port=41
  AMK_Motor_temp_RL : Outport  Port=42
  AMK_Motor_temp_RR : Outport  Port=43
  AMK_INV_temp_FL : Outport  Port=44
  AMK_INV_temp_FR : Outport  Port=45
  AMK_INV_temp_RL : Outport  Port=46
  AMK_INV_temp_RR : Outport  Port=47
  wires:
  Gain7/1 -> Gain9/1
  Read CM Dict24/1 -> Gain7/1
  Read CM Dict25/1 -> Gain10/1
  Gain10/1 -> Gain11/1
  Gain12/1 -> Gain13/1
  Gain14/1 -> Gain15/1
  Read CM Dict26/1 -> Gain12/1
  Read CM Dict27/1 -> Gain14/1
  Gain9/1 -> Data Type Conversion11/1  "Motor_RPM"
  Gain15/1 -> Data Type Conversion12/1  "Motor_RPM"
  Gain13/1 -> Data Type Conversion13/1  "Motor_RPM"
  Gain11/1 -> Data Type Conversion14/1  "Motor_RPM"
  Data Type Conversion11/1 -> RPM scope/1, RPM_FL/1
  Data Type Conversion14/1 -> RPM scope/2, RPM_FR/1
  Data Type Conversion13/1 -> RPM scope/3, RPM_RL/1
  Data Type Conversion12/1 -> RPM scope/4, RPM_RR/1
  Read CM Dict12/1 -> Data Type Conversion15/1
  Data Type Conversion15/1 -> Scope/1
  Read CM Dict15/1 -> Data Type Conversion18/1
  Data Type Conversion18/1 -> KERS_pos/1, BPS/1, Gain/1, "Brake "/1
  Data Type Conversion19/1 -> TPS/1, "Throttle "/1
  Constant1/1 -> Data Type Conversion21/1
  Constant2/1 -> Data Type Conversion20/1
  Constant3/1 -> Data Type Conversion22/1
  Constant4/1 -> Data Type Conversion23/1
  Data Type Conversion25/1 -> damper_rate_FL/1
  Discrete Derivative4/1 -> Data Type Conversion25/1
  Data Type Conversion24/1 -> damper_rate_FR/1
  Discrete Derivative5/1 -> Data Type Conversion24/1
  Data Type Conversion26/1 -> damper_rate_RL/1
  Discrete Derivative6/1 -> Data Type Conversion26/1
  Data Type Conversion27/1 -> damper_rate_RR/1
  Discrete Derivative7/1 -> Data Type Conversion27/1
  Read CM Dict20/1 -> Data Type Conversion47/1
  Read CM Dict21/1 -> Data Type Conversion48/1
  Data Type Conversion47/1 -> steering wheel angle/1, "Steering_wheel_angle "/1
  Data Type Conversion48/1 -> Steering_wheel_speed/1
  Data Type Conversion17/1 -> DC_voltage/1
  Constant21/1 -> Data Type Conversion17/1
  Read CM Dict30/1 -> Gain29/1
  Read CM Dict31/1 -> Gain30/1
  Read CM Dict32/1 -> Gain31/1
  Read CM Dict29/1 -> Gain28/1
  Data Type Conversion43/1 -> Damper pos/2, damper_pos_FR/1
  Data Type Conversion45/1 -> Damper pos/3, damper_pos_RL/1
  Data Type Conversion44/1 -> Damper pos/1, damper_pos_FL/1
  Data Type Conversion46/1 -> Damper pos/4, damper_pos_RR/1
  Sum/1 -> Saturation/1
  Gain30/1 -> Sum2/1
  Gain31/1 -> Sum3/1
  correctionConstantRear/1 -> Sum3/2, Sum2/2
  Sum1/1 -> Saturation1/1
  Sum2/1 -> Saturation2/1
  Sum3/1 -> Saturation3/1
  Saturation/1 -> Data Type Conversion44/1
  Saturation1/1 -> Data Type Conversion43/1
  Saturation2/1 -> Data Type Conversion45/1
  Saturation3/1 -> Data Type Conversion46/1
  Read CM Dict33/1 -> Discrete Derivative4/1
  Read CM Dict34/1 -> Discrete Derivative5/1
  Read CM Dict35/1 -> Discrete Derivative6/1
  Read CM Dict36/1 -> Discrete Derivative7/1
  Data Type Conversion30/1 -> AMK_INV_temp_FL/1
  Constant5/1 -> Data Type Conversion30/1
  Data Type Conversion54/1 -> AMK_Motor_temp_FL/1
  Constant6/1 -> Data Type Conversion54/1
  Data Type Conversion2/1 -> AMK_Motor_temp_FR/1
  Constant7/1 -> Data Type Conversion2/1
  Data Type Conversion3/1 -> AMK_Motor_temp_RL/1
  Constant8/1 -> Data Type Conversion3/1
  Data Type Conversion4/1 -> AMK_Motor_temp_RR/1
  Constant18/1 -> Data Type Conversion4/1
  Data Type Conversion5/1 -> AMK_INV_temp_FR/1
  Constant19/1 -> Data Type Conversion5/1
  Data Type Conversion28/1 -> AMK_INV_temp_RL/1
  Constant20/1 -> Data Type Conversion28/1
  Data Type Conversion29/1 -> AMK_INV_temp_RR/1
  Constant22/1 -> Data Type Conversion29/1
  Data Type Conversion33/1 -> Iq/1, Iq_FL/1
  Data Type Conversion37/1 -> Iq/2, Iq_FR/1
  Data Type Conversion38/1 -> Iq/3, Iq_RL/1
  Data Type Conversion39/1 -> Iq/4, Iq_RR/1
  Constant11/1 -> Data Type Conversion37/1
  Constant12/1 -> Data Type Conversion38/1
  Constant13/1 -> Data Type Conversion39/1
  Constant9/1 -> Data Type Conversion33/1
  Data Type Conversion32/1 -> Id/1, Id_FL/1
  Data Type Conversion40/1 -> Id/2, Id_FR/1
  Data Type Conversion41/1 -> Id/3, Id_RL/1
  Data Type Conversion42/1 -> Id/4, Id_RR/1
  Constant16/1 -> Data Type Conversion42/1
  Constant14/1 -> Data Type Conversion40/1
  Constant15/1 -> Data Type Conversion41/1
  Constant10/1 -> Data Type Conversion32/1
  Discrete Derivative1/1 -> "RPM_Der_scope "/2, RPM_der_FR/1
  Discrete Derivative2/1 -> "RPM_Der_scope "/3, RPM_der_RL/1
  Discrete Derivative3/1 -> "RPM_Der_scope "/4, RPM_der_RR/1
  Gain21/1 -> Data Type Conversion50/1  "Motor_RPM"
  Gain23/1 -> Data Type Conversion49/1  "Motor_RPM"
  Gain26/1 -> Gain27/1
  Gain25/1 -> Data Type Conversion52/1  "Motor_RPM"
  Data Type Conversion51/1 -> Discrete Derivative2/1
  Gain27/1 -> Data Type Conversion51/1  "Motor_RPM"
  Data Type Conversion52/1 -> Discrete Derivative1/1
  Data Type Conversion50/1 -> Discrete Derivative3/1
  Gain20/1 -> Gain21/1
  Gain24/1 -> Gain25/1
  Gain22/1 -> Gain23/1
  Read CM Dict22/1 -> Gain22/1
  Read CM Dict28/1 -> Gain26/1
  Read CM Dict14/1 -> Gain20/1
  Read CM Dict23/1 -> Gain24/1
  Data Type Conversion10/1 -> roll rate/1, roll_rate/1
  Data Type Conversion9/1 -> Gain1/1, roll_angle/1
  Data Type Conversion/1 -> V_x_INS/1, Vx_INS_Scope/1
  Data Type Conversion1/1 -> V_y_INS/1
  Data Type Conversion6/1 -> yawRate/1, YawRate_INS/1
  Data Type Conversion16/1 -> yawRate_der/1
  Data Type Conversion7/1 -> ay/1
  Data Type Conversion8/1 -> "ax "/1
  Read CM Dict2/1 -> Ay_Ax_INS/1, Sum6/1
  Read CM Dict9/1 -> Sum7/1, Ay_Ax_INS/2
  Read CM Dict13/1 -> Data Type Conversion16/1
  Read CM Dict11/1 -> Data Type Conversion10/1
  Read CM Dict10/1 -> Data Type Conversion9/1
  Read CM Dict8/1 -> Data Type Conversion1/1
  Read CM Dict7/1 -> Data Type Conversion/1
  Read CM Dict1/1 -> Data Type Conversion6/1
  "estimated \"Measured Power\" based on Torque, RPM and datasheet IRL this is measured"/1(Out2) -> power/1
  Gain1/1 -> "roll angle "/1
  Gain28/1 -> Sum/2
  Gain29/1 -> Sum1/2
  correctionCornstantFront/1 -> Sum/1, Sum1/1
  Gain/1 -> TPS/2
  Band-Limited White Noise/1 -> Rate Transition19/1
  Rate Transition19/1 -> ?
  Sum4/1 -> Data Type Conversion19/1
  Read CM Dict/1 -> Sum4/1
  Band-Limited White Noise1/1 -> Rate Transition1/1
  Band-Limited White Noise2/1 -> Rate Transition2/1
  Sum6/1 -> Data Type Conversion7/1
  Band-Limited White Noise3/1 -> Rate Transition3/1
  Sum7/1 -> Data Type Conversion8/1
  Rate Transition1/1 -> Gain2/1
  Rate Transition2/1 -> ?
  Data Type Conversion49/1 -> Discrete Derivative8/1
  Discrete Derivative8/1 -> "RPM_Der_scope "/1, RPM_der_FL/1

== system TV_2018_HIL/CarMaker/Function-Call Subsystem4 ==
  CAN_MSG : Inport
  function : TriggerPort  TriggerType=function-call  VariantControl=Variant
  AMK Inverter Setpoints from ECU : Subsystem
  CAN Pack27 : canmsglib/CAN Pack  MsgList=(none)  MsgName=CAN Msg  MsgIDType=Standard (11-bit identifier)  MsgIdentifier=DRIVE_ENABLE  MsgLength=0  NSignals=0  StartBits=0  SignalSizes=0  ByteOrders=0  DataTypes=0  MultiplexTypes=0  MultiplexValues=0  Factors=0  Offsets=0  Minimums=0  Maximums=0  Remote=off
      settings: DataFormat=manually specified signals
  CAN Transmit27 : canlib/CAN Transmit  BlockHandle=3058.0002  DeviceMenu=Kvaser Virtual 1 (Channel 1)  Device=PEAK-System PCAN-USB (PCAN_USBBUS1)  ObjConstructor=canChannel('PEAK-System', 'PCAN_PCIBUS1')  EnablePeriodicTransmit=off  MessagePeriod=1.000
  CAN Unpack1 : canmsglib/CAN Unpack  MsgList=(none)  MsgName=ECU_SET_POINT_FR_ID  MsgIDType=Standard (11-bit identifier)  MsgIdentifier=ECU_SET_POINT_FR_ID  MsgLength=6  SignalInfo=trq_pos$0$16$1$1$1$0$1$0$-Inf$Inf$#trq_neg$16$16$1$1$1$0$1$0$-Inf$Inf$#w_set$32$16$1$1$1$0$1$0$-Inf$Inf$#  NSignals=3  IDPort=off  TimestampPort=on  ErrorPort=off  RemotePort=off  LengthPort=off  StatusPort=off  StartBits=str2num('[int32(0);int32(16);int32(32)]')  SignalSizes=str2num('[int32(16);int32(16);int32(16)]')  ByteOrders=str2num('[int32(1);int32(1);int32(1)]')  DataTypes=str2num('[int32(1);int32(1);int32(1)]')  MultiplexTypes=str2num('[int32(1);int32(1);int32(1)]')  MultiplexValues=str2num('[double(0);double(0);double(0)]')  Factors=str2num('[double(1);double(1);double(1)]')  Offsets=str2num('[double(0);double(0);double(0)]')  Minimums=str2num('[double(-Inf);double(-Inf);double(-Inf)]')  Maximums=str2num('[double(Inf);double(Inf);double(Inf)]')
  CAN Unpack2 : canmsglib/CAN Unpack  MsgList=(none)  MsgName=ECU_SET_POINT_RL_ID  MsgIDType=Standard (11-bit identifier)  MsgIdentifier=ECU_SET_POINT_RL_ID  MsgLength=6  SignalInfo=trq_pos$0$16$1$1$1$0$1$0$-Inf$Inf$#trq_neg$16$16$1$1$1$0$1$0$-Inf$Inf$#w_set$32$16$1$1$1$0$1$0$-Inf$Inf$#  NSignals=3  IDPort=off  TimestampPort=on  ErrorPort=off  RemotePort=off  LengthPort=off  StatusPort=off  StartBits=str2num('[int32(0);int32(16);int32(32)]')  SignalSizes=str2num('[int32(16);int32(16);int32(16)]')  ByteOrders=str2num('[int32(1);int32(1);int32(1)]')  DataTypes=str2num('[int32(1);int32(1);int32(1)]')  MultiplexTypes=str2num('[int32(1);int32(1);int32(1)]')  MultiplexValues=str2num('[double(0);double(0);double(0)]')  Factors=str2num('[double(1);double(1);double(1)]')  Offsets=str2num('[double(0);double(0);double(0)]')  Minimums=str2num('[double(-Inf);double(-Inf);double(-Inf)]')  Maximums=str2num('[double(Inf);double(Inf);double(Inf)]')
  CAN Unpack3 : canmsglib/CAN Unpack  MsgList=(none)  MsgName=ECU_SET_POINT_RR_ID  MsgIDType=Standard (11-bit identifier)  MsgIdentifier=ECU_SET_POINT_RR_ID  MsgLength=6  SignalInfo=trq_pos$0$16$1$1$1$0$1$0$-Inf$Inf$#trq_neg$16$16$1$1$1$0$1$0$-Inf$Inf$#w_set$32$16$1$1$1$0$1$0$-Inf$Inf$#  NSignals=3  IDPort=off  TimestampPort=on  ErrorPort=off  RemotePort=off  LengthPort=off  StatusPort=off  StartBits=str2num('[int32(0);int32(16);int32(32)]')  SignalSizes=str2num('[int32(16);int32(16);int32(16)]')  ByteOrders=str2num('[int32(1);int32(1);int32(1)]')  DataTypes=str2num('[int32(1);int32(1);int32(1)]')  MultiplexTypes=str2num('[int32(1);int32(1);int32(1)]')  MultiplexValues=str2num('[double(0);double(0);double(0)]')  Factors=str2num('[double(1);double(1);double(1)]')  Offsets=str2num('[double(0);double(0);double(0)]')  Minimums=str2num('[double(-Inf);double(-Inf);double(-Inf)]')  Maximums=str2num('[double(Inf);double(Inf);double(Inf)]')
  CAN Unpack4 : canmsglib/CAN Unpack  MsgList=(none)  MsgName=TestTimestamp  MsgIDType=Standard (11-bit identifier)  MsgIdentifier=9  MsgLength=4  SignalInfo=timestamp$0$32$1$2$1$0$1$0$-Inf$Inf$#  NSignals=1  IDPort=off  TimestampPort=on  ErrorPort=off  RemotePort=off  LengthPort=off  StatusPort=off  StartBits=str2num('[int32(0)]')  SignalSizes=str2num('[int32(32)]')  ByteOrders=str2num('[int32(1)]')  DataTypes=str2num('[int32(2)]')  MultiplexTypes=str2num('[int32(1)]')  MultiplexValues=str2num('[double(0)]')  Factors=str2num('[double(1)]')  Offsets=str2num('[double(0)]')  Minimums=str2num('[double(-Inf)]')  Maximums=str2num('[double(Inf)]')
  CAN Unpack5 : canmsglib/CAN Unpack  MsgList=(none)  MsgName=SlipRatios  MsgIDType=Standard (11-bit identifier)  MsgIdentifier=200  MsgLength=8  SignalInfo=SR_FL$0$16$1$1$1$0$1$0$-Inf$Inf$#SR_FR$16$16$1$1$1$0$1$0$-Inf$Inf$#SR_RL$32$16$1$1$1$0$1$0$-Inf$Inf$#SR_RR$48$16$1$1$1$0$1$0$-Inf$Inf$#  NSignals=4  IDPort=off  TimestampPort=on  ErrorPort=off  RemotePort=off  LengthPort=off  StatusPort=off  StartBits=str2num('[int32(0);int32(16);int32(32);int32(48)]')  SignalSizes=str2num('[int32(16);int32(16);int32(16);int32(16)]')  ByteOrders=str2num('[int32(1);int32(1);int32(1);int32(1)]')  DataTypes=str2num('[int32(1);int32(1);int32(1);int32(1)]')  MultiplexTypes=str2num('[int32(1);int32(1);int32(1);int32(1)]')  MultiplexValues=str2num('[double(0);double(0);double(0);double(0)]')  Factors=str2num('[double(1);double(1);double(1);double(1)]')  Offsets=str2num('[double(0);double(0);double(0);double(0)]')  Minimums=str2num('[double(-Inf);double(-Inf);double(-Inf);double(-Inf)]')  Maximums=str2num('[double(Inf);double(Inf);double(Inf);double(Inf)]')
  CAN Unpack6 : canmsglib/CAN Unpack  MsgList=(none)  MsgName=yawRatefeed  MsgIDType=Standard (11-bit identifier)  MsgIdentifier=201  MsgLength=2  SignalInfo=yawRate$0$16$1$1$1$0$1$0$-Inf$Inf$#  NSignals=1  IDPort=off  TimestampPort=on  ErrorPort=off  RemotePort=off  LengthPort=off  StatusPort=off  StartBits=str2num('[int32(0)]')  SignalSizes=str2num('[int32(16)]')  ByteOrders=str2num('[int32(1)]')  DataTypes=str2num('[int32(1)]')  MultiplexTypes=str2num('[int32(1)]')  MultiplexValues=str2num('[double(0)]')  Factors=str2num('[double(1)]')  Offsets=str2num('[double(0)]')  Minimums=str2num('[double(-Inf)]')  Maximums=str2num('[double(Inf)]')
  CAN Unpack7 : canmsglib/CAN Unpack  MsgList=(none)  MsgName=TestTimestamp  MsgIDType=Standard (11-bit identifier)  MsgIdentifier=ECU_FZ_DAMPER_EST_ID  MsgLength=8  SignalInfo=FL_z$0$16$1$2$1$0$1$0$-Inf$Inf$#FR_z$16$16$1$1$1$0$1$0$-Inf$Inf$#RL_z$32$16$1$1$1$0$1$0$-Inf$Inf$#RR_z$48$16$1$1$1$0$1$0$-Inf$Inf$#  NSignals=4  IDPort=off  TimestampPort=on  ErrorPort=off  RemotePort=off  LengthPort=off  StatusPort=off  StartBits=str2num('[int32(0);int32(16);int32(32);int32(48)]')  SignalSizes=str2num('[int32(16);int32(16);int32(16);int32(16)]')  ByteOrders=str2num('[int32(1);int32(1);int32(1);int32(1)]')  DataTypes=str2num('[int32(2);int32(1);int32(1);int32(1)]')  MultiplexTypes=str2num('[int32(1);int32(1);int32(1);int32(1)]')  MultiplexValues=str2num('[double(0);double(0);double(0);double(0)]')  Factors=str2num('[double(1);double(1);double(1);double(1)]')  Offsets=str2num('[double(0);double(0);double(0);double(0)]')  Minimums=str2num('[double(-Inf);double(-Inf);double(-Inf);double(-Inf)]')  Maximums=str2num('[double(Inf);double(Inf);double(Inf);double(Inf)]')
  CAN Unpack8 : canmsglib/CAN Unpack  MsgList=(none)  MsgName=TestTimestamp  MsgIDType=Standard (11-bit identifier)  MsgIdentifier=ECU_ALIVE_ID  MsgLength=1  SignalInfo=Alive$0$8$1$2$1$0$1$0$-Inf$Inf$#  NSignals=1  IDPort=off  TimestampPort=on  ErrorPort=off  RemotePort=off  LengthPort=off  StatusPort=off  StartBits=str2num('[int32(0)]')  SignalSizes=str2num('[int32(8)]')  ByteOrders=str2num('[int32(1)]')  DataTypes=str2num('[int32(2)]')  MultiplexTypes=str2num('[int32(1)]')  MultiplexValues=str2num('[double(0)]')  Factors=str2num('[double(1)]')  Offsets=str2num('[double(0)]')  Minimums=str2num('[double(-Inf)]')  Maximums=str2num('[double(Inf)]')
  CAN Unpack9 : canmsglib/CAN Unpack  MsgList=(none)  MsgName=TestTimestamp  MsgIDType=Standard (11-bit identifier)  MsgIdentifier=DRIVE_ENABLE  MsgLength=1  SignalInfo=Alive$0$8$1$2$1$0$1$0$-Inf$Inf$#  NSignals=1  IDPort=off  TimestampPort=on  ErrorPort=off  RemotePort=off  LengthPort=off  StatusPort=off  StartBits=str2num('[int32(0)]')  SignalSizes=str2num('[int32(8)]')  ByteOrders=str2num('[int32(1)]')  DataTypes=str2num('[int32(2)]')  MultiplexTypes=str2num('[int32(1)]')  MultiplexValues=str2num('[double(0)]')  Factors=str2num('[double(1)]')  Offsets=str2num('[double(0)]')  Minimums=str2num('[double(-Inf)]')  Maximums=str2num('[double(Inf)]')
  CAN_SR : Scope
  Fi_z from ECU : Scope  NumInputPorts=4
  Gain{,1..3} (4 alike) : Gain  Gain=1/1000
  Gain4 : Gain  Gain=single(0.01)
  Memory : Memory  InheritSampleTime=on
  Mux : Mux
  Mux1 : Mux
  Scope{,7,9..11,13,15} (7 alike) : Scope
  Sum : Sum  Inputs=|-+
  To File : ToFile  Filename=Mat_files_CAN\Can_timestamps.mat  MatrixName=ts  SaveFormat=Timeseries
  To File1 : ToFile  Filename=Mat_files_CAN\testTs.mat  MatrixName=testTs
  To File2 : ToFile  Filename=Mat_files_CAN\Can_SR  MatrixName=sr  SaveFormat=Timeseries
  To File3 : ToFile  Filename=Mat_files_CAN\yawRateRef.mat  MatrixName=rRef  SaveFormat=Timeseries
  yawRateref : Scope
  timestampFL : Outport
  testTs : Outport  Port=2
  wires:
  CAN Unpack3/3 -> ?
  [A] -> Sum/2, Scope13/1, Memory/1, Mux/1  "t_FL"
  Mux/1 -> To File/1, Scope7/1
  CAN Unpack4/1 -> testTs/1, Scope9/1, To File1/1
  CAN Unpack4/2 -> Scope10/1
  Sum/1 -> Scope11/1, timestampFL/1
  Memory/1 -> Sum/1
  CAN Unpack5/1 -> Gain/1
  Mux1/1 -> CAN_SR/1, To File2/1
  CAN Unpack5/2 -> Gain1/1
  CAN Unpack5/3 -> Gain2/1
  CAN Unpack5/4 -> Gain3/1
  Gain/1 -> Mux1/1
  Gain1/1 -> Mux1/2
  Gain2/1 -> Mux1/3
  Gain3/1 -> Mux1/4
  CAN Unpack6/1 -> Scope15/1, Gain4/1
  Gain4/1 -> yawRateref/1, To File3/1
  [B] -> Mux/2
  [C] -> Mux/3
  [D] -> Mux/4
  CAN_MSG/1 -> CAN Unpack8/1, CAN Unpack9/1, AMK Inverter Setpoints from ECU/1(In1), AMK Inverter Setpoints from ECU/5(In5), AMK Inverter Setpoints from ECU/6(In6), CAN Unpack7/1, CAN Unpack6/1, CAN Unpack5/1, CAN Unpack4/1, AMK Inverter Setpoints from ECU/2(In2)
  CAN Unpack7/1 -> Fi_z from ECU/1
  CAN Unpack7/2 -> Fi_z from ECU/2
  CAN Unpack7/3 -> Fi_z from ECU/3
  CAN Unpack7/4 -> Fi_z from ECU/4
  CAN Unpack8/1 -> Scope/1

== system TV_2018_HIL/CarMaker/IPG Vehicle3 ==
  Sync_In : Inport
  Vhcl.Model.Source : Inport  Port=2
  VhclCtrl.Steering : Inport  Port=3
  Vhcl.Wheel.In : Inport  Port=4
  Vhcl.Misc : Inport  Port=5
  VhclCtrl.Brake : Inport  Port=6
  VhclCtrl.PT : Inport  Port=7
  Brake : Subsystem
  CarAndTrailer : Subsystem
  PowerTrain : Subsystem
  Stop Simulation : Stop
  VehicleSource_BuiltIn : simulink/Logic and Bit Operations/Compare To Constant  relop=~=  const=1  OutDataTypeStr=boolean  ZeroCross=off
  Sync_Out : Outport
  wires:
  VhclCtrl.PT/1 -> PowerTrain/3(VhclCtrl.PT)
  Brake/1(Sync_Out) -> PowerTrain/1(Sync_In)
  CarAndTrailer/1(Sync_Out) -> Brake/1(Sync_In)
  CarAndTrailer/2(Brake.IF.In) -> Brake/2(Brake.IF.In)
  VhclCtrl.Brake/1 -> Brake/3(VhclCtrl.Brake)
  PowerTrain/1(Sync_Out) -> Sync_Out/1
  Vhcl.Misc/1 -> CarAndTrailer/4(Vhcl.Misc)
  Vhcl.Wheel.In/1 -> CarAndTrailer/3(Vhcl.Wheel.In)
  VhclCtrl.Steering/1 -> CarAndTrailer/2(VhclCtrl.Steering)
  Sync_In/1 -> CarAndTrailer/1(Sync_In)
  Vhcl.Model.Source/1 -> VehicleSource_BuiltIn/1
  VehicleSource_BuiltIn/1 -> Stop Simulation/1
  Brake/2(Vhcl.Wheel.PT) -> PowerTrain/2(Vhcl.Wheel.PT)

== system TV_2018_HIL/CarMaker/Open GUI ==
  S-Function : S-Function  FunctionName=cm_gui  SFunctionDeploymentMode=off  EnableBusSupport=off
